simulink model "DiscreteControlRTS"  (R2022a)
settings: Solver=FixedStepAuto  StartTime=0.0  StopTime=30  FixedStep=10/1000  RelTol=1e-3  EnableMultiTasking=on
values from neighbouring files (symbols this model uses):
  coeff_R = sym2poly(R(z))    [RTS.m]
  coeff_S = sym2poly(S(z))    [RTS.m]
  coeff_T = sym2poly(T(z))    [RTS.m]
undefined symbols (not defined in the file or in its folder): Az, Bz
settings Model: Creator=g.reynosomeza  LastModifiedBy=natha
settings SolverCC: AlgebraicLoopSolver=TrustRegion
settings DataIOCC: LimitDataPoints=on  SaveFormat=Array  ReturnWorkspaceOutputs=off
settings OptimizationCC: LifeSpan=inf
settings DebuggingCC: AlgebraicLoopMsg=none  ArtificialAlgebraicLoopMsg=none  SolverPrmCheckMsg=warning  UnconnectedInputMsg=warning  UnconnectedOutputMsg=warning  UnconnectedLineMsg=warning  SFUnexpectedBacktrackingDiag=warning  SFNoUnconditionalDefaultTransitionDiag=warning  SFMachineParentedDataDiag=warning  ArithmeticOperatorsInVariantConditions=warning
settings HardwareCC: ProdBitPerPointer=32  ProdBitPerSizeT=32  ProdBitPerPtrDiffT=32  ProdLargestAtomicFloat=None  ProdIntDivRoundTo=Undefined  ProdEndianess=Unspecified  ProdWordSize=32  ProdHWDeviceType=32-bit Generic
settings ModelReferenceCC: PropagateSignalLabelsOutOfModel=off
settings SFSimCC: SimUseLocalCustomCode=off  CustomCodeUndefinedFunction=UseInterfaceOnly
settings RTWCC: RTWUseLocalCustomCode=off  DLArmComputeVersion=19.05
settings CodeAppCC: StateflowObjectComments=on
settings GRTTargetCC: TargetLangStandard=C89/C90 (ANSI)
settings ConfigComp: CovMetricSettings=dw  CovSaveCumulativeToWorkspaceVar=on  CovSaveSingleToWorkspaceVar=on  CovExternalEMLEnable=off  CovSFcnEnable=off

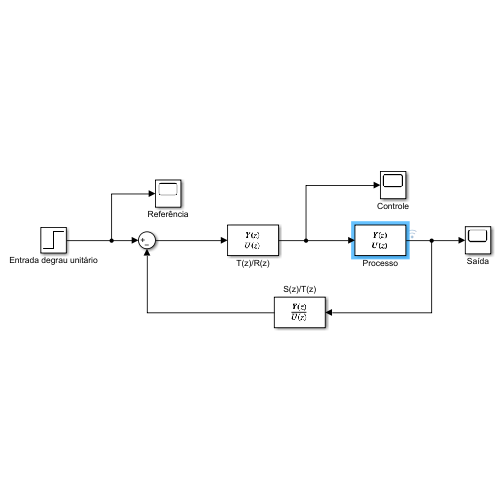
[thumbnail: Simulink's stored preview of the top-level diagram]
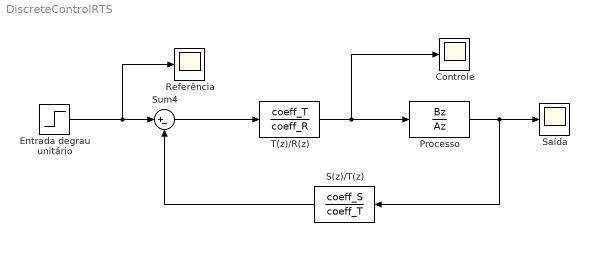
== system DiscreteControlRTS ==
  Controle : Scope
  Entrada degrau unitário : Step  Time=0  SampleTime=0.25
  Processo : DiscreteTransferFcn  Numerator=Bz  Denominator=Az
  Referência : Scope
  S(z)/T(z) : DiscreteTransferFcn  Numerator=coeff_S  Denominator=coeff_T
  Saída : Scope
  Sum4 : Sum  Inputs=|+-
  T(z)/R(z) : DiscreteTransferFcn  Numerator=coeff_T  Denominator=coeff_R
  wires:
  T(z)/R(z)/1 -> Processo/1, Controle/1
  Entrada degrau unitário/1 -> Referência/1, Sum4/1
  Processo/1 -> Saída/1, S(z)/T(z)/1
  Sum4/1 -> T(z)/R(z)/1
  S(z)/T(z)/1 -> Sum4/2
